simulink model "realtime_motor"  (R2024b)
settings: Solver=ode5  StartTime=0.0  StopTime=20  FixedStep=0.001  RelTol=1e-3
InitFcn:
  | Init
values from neighbouring files (symbols this model uses):
  Beq = (Beq_hat_pos + Beq_hat_neg)/2    [Parameters_estimation.m]    (also in Real_time_parameter_estimation.m = (data.Beq_hat_pos + data.Beq_hat_neg)/2; real-time-estimation.mat = 9.67900035512e-07)
  delta_est = 1/sqrt(2)    [Init.m]
  tau_sf = (abs(tau_sf_pos)+abs(tau_sf_neg))/2    [Parameters_estimation.m]    (also in Real_time_parameter_estimation.m = (abs(data.tau_sf_pos)+abs(data.tau_sf_neg))/2; real-time-estimation.mat = 0.00454084382337)
  wc = 2*pi*20    (= 125.663706144)    [Init.m]
undefined symbols (not defined in the file or in its folder): degs2rpm, gbox, Kd, Ki, Kp, mot, National_Instruments, PCI, rpm2degs, rpm2rads, sens, tl
libraries: sldrtlib x3, simulink x2
settings Model: SimulationMode=external  ExtModeTrigDuration=1000001  Creator=galeazzolu  LastModifiedBy=galeazzolu
settings DataIOCC: ReturnWorkspaceOutputs=off
settings HardwareCC: ProdBitPerLong=64  ProdHWDeviceType=Intel->x86-64 (Linux 64)
settings RTWCC: Description=Simulink Desktop Real-Time  SystemTargetFile=sldrt.tlc  TemplateMakefile=sldrt.tmf  RTWCompilerOptimization=on
settings CodeAppCC: MaxIdLength=95
settings SimulinkDesktopRealTimeCC: TargetLibSuffix=_sldrt.a  TargetPreCompLibLocation=C:\Program Files\MATLAB\R2024b\toolbox\sldrt\lib\win64  ParMdlRefBuildCompliant=on

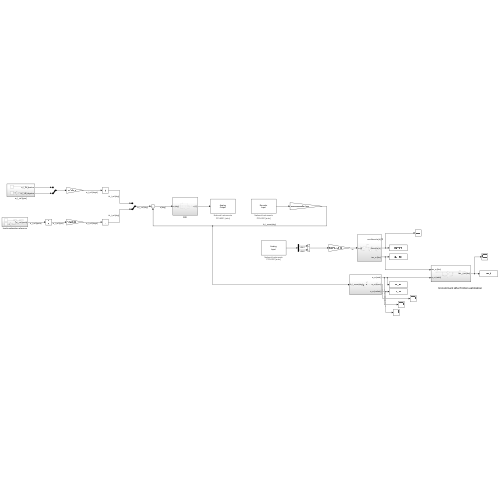
[thumbnail: Simulink's stored preview of the top-level diagram]
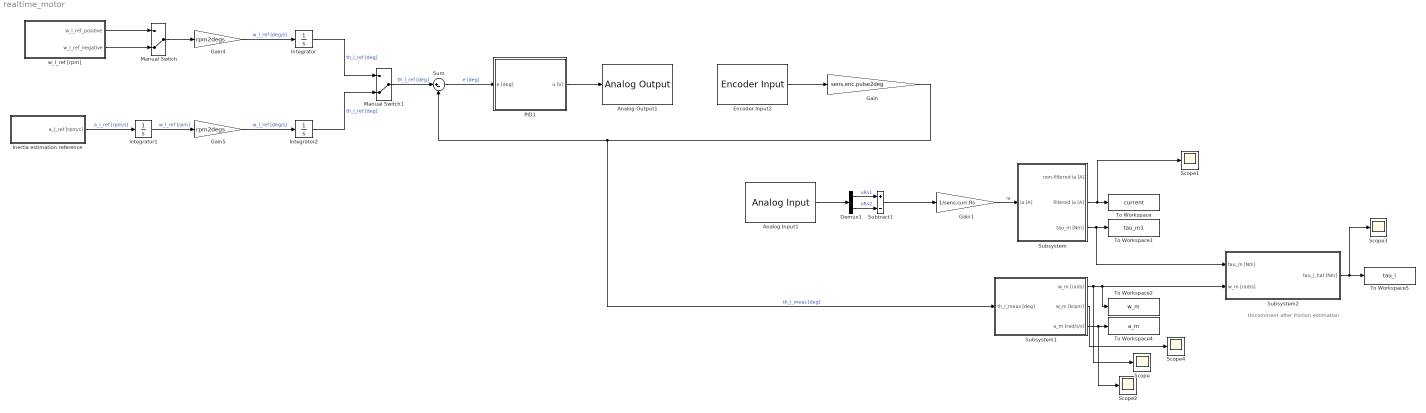
== system realtime_motor ==
  note: Uncomment after friction estimation
  Analog Input1 : sldrtlib/Analog Input  SampleTime=-1  MaxMissedTicks=10  ShowMissedTicks=off  YieldWhenWaiting=off  DrvName=National_Instruments/PCI-6221  DrvAddress=4294967295  DrvOptions=[0 0 0 2 0]  Channels=[1,2]  RangeMode=1  VoltRange=1  DataType=1
      settings: AttributesFormatString=National Instruments\nPCI-6221 [auto]
  Analog Output1 : sldrtlib/Analog Output  SampleTime=-1  MaxMissedTicks=10  ShowMissedTicks=off  YieldWhenWaiting=off  DrvName=National_Instruments/PCI-6221  DrvAddress=4294967295  DrvOptions=[0 0 0 2 0]  Channels=1  RangeMode=1  VoltRange=1  InitialValue=0  FinalValue=0
      settings: AttributesFormatString=National Instruments\nPCI-6221 [auto]
  Demux1 : Demux  Outputs=2
  Encoder Input2 : sldrtlib/Encoder Input  SampleTime=-1  MaxMissedTicks=10  ShowMissedTicks=off  YieldWhenWaiting=off  DrvName=National_Instruments/PCI-6221  DrvAddress=4294967295  DrvOptions=[0 0 0 2 0]  Channels=1  QuadMode=3  IndexPulse=1  InputFilter=Inf  DataType=1
      settings: AttributesFormatString=National Instruments\nPCI-6221 [auto]
  Gain : Gain  Gain=sens.enc.pulse2deg
  Gain1 : Gain  Gain=1/sens.curr.Rs
  Gain4 : Gain  Gain=rpm2degs
  Gain5 : Gain  Gain=rpm2degs
  Inertia estimation reference : Subsystem
  Integrator : Integrator
  Integrator1 : Integrator
  Integrator2 : Integrator
  Manual Switch : ManualSwitch  CurrentSetting=0
  Manual Switch1 : ManualSwitch  CurrentSetting=0
  PID1 : Subsystem
  Scope{,1..4} (5 alike) : Scope
  Subsystem : Subsystem
  Subsystem1 : Subsystem
  Subsystem2 : Subsystem
  Subtract1 : Sum  Inputs=+-
  Sum : Sum  Inputs=|+-
  To Workspace : ToWorkspace  VariableName=current  SaveFormat=Structure With Time  SampleTime=-1
  To Workspace1 : ToWorkspace  VariableName=tau_m1  SaveFormat=Structure With Time  SampleTime=-1
  To Workspace2 : ToWorkspace  VariableName=w_m  SaveFormat=Structure With Time  SampleTime=-1
  To Workspace4 : ToWorkspace  VariableName=a_m  SaveFormat=Structure With Time  SampleTime=-1
  To Workspace5 : ToWorkspace  VariableName=tau_i  SaveFormat=Structure With Time  SampleTime=-1
  w_l_ref [rpm] : Subsystem
  wires:
  Integrator1/1 -> Gain5/1  "w_l_ref [rpm]"
  w_l_ref [rpm]/1(w_l_ref_positive) -> Manual Switch/1
  Integrator2/1 -> Manual Switch1/2  "th_l_ref [deg]"
  Subsystem1/2(w_m [krpm]) -> Scope4/1
  Subsystem/2(filtered ia [A]) -> Scope1/1, To Workspace/1
  Manual Switch1/1 -> Sum/1  "th_l_ref [deg]"
  Sum/1 -> PID1/1(e [deg])  "e [deg]"
  PID1/1(u [V]) -> Analog Output1/1
  w_l_ref [rpm]/2(w_l_ref_negative) -> Manual Switch/2
  Gain/1 -> Subsystem1/1(th_l_meas [deg]), Sum/2  "th_l_meas [deg]"
  Demux1/1 -> Subtract1/1  "uRs1"
  Subsystem/3(tau_m [Nm]) -> Subsystem2/1(tau_m [Nm]), To Workspace1/1
  Gain4/1 -> Integrator/1  "w_l_ref [deg/s]"
  Gain1/1 -> Subsystem/1(ia [A])  "ia"
  Subsystem1/1(w_m [rads]) -> Subsystem2/2(w_m [rad/s]), To Workspace2/1, Scope/1
  Manual Switch/1 -> Gain4/1
  Demux1/2 -> Subtract1/2  "uRs2"
  Subsystem2/1(tau_i_hat [Nm]) -> Scope3/1, To Workspace5/1
  Integrator/1 -> Manual Switch1/1  "th_l_ref [deg]"
  Subtract1/1 -> Gain1/1
  Gain5/1 -> Integrator2/1  "w_l_ref [deg/s]"
  Inertia estimation reference/1(a_l_ref [rpm/s]) -> Integrator1/1  "a_l_ref [rpm/s]"
  Subsystem1/3(a_m [rad/s/s]) -> Scope2/1, To Workspace4/1
  Encoder Input2/1 -> Gain/1
  Analog Input1/1 -> Demux1/1

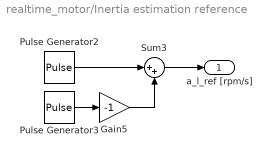
== system realtime_motor/Inertia estimation reference ==
  Gain5 : Gain  Gain=-1
  Pulse Generator2 : DiscretePulseGenerator  PulseType=Time based  Amplitude=450  PulseWidth=50
  Pulse Generator3 : DiscretePulseGenerator  PulseType=Time based  Amplitude=450  PulseWidth=50  PhaseDelay=1
  Sum3 : Sum  Inputs=|++
  a_l_ref [rpm/s] : Outport
  wires:
  Pulse Generator3/1 -> Gain5/1
  Pulse Generator2/1 -> Sum3/1
  Gain5/1 -> Sum3/2
  Sum3/1 -> a_l_ref [rpm/s]/1

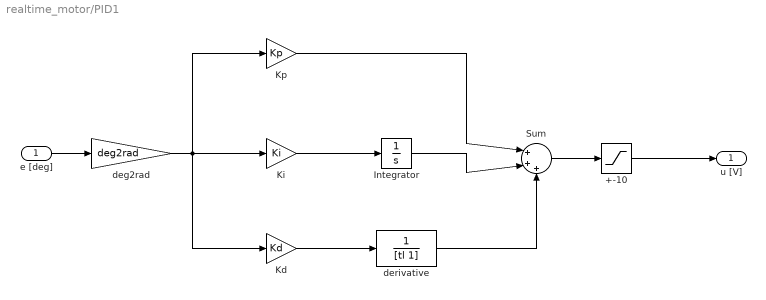
== system realtime_motor/PID1 ==
  e [deg] : Inport
  +-10 : Saturate  UpperLimit=10  LowerLimit=-10
  Integrator : Integrator
  Kd : Gain  Gain=Kd
  Ki : Gain  Gain=Ki
  Kp : Gain  Gain=Kp
  Sum : Sum  Inputs=|+++
  deg2rad : Gain  Gain=deg2rad
  derivative : TransferFcn  Denominator=[tl 1]
  u [V] : Outport
  wires:
  e [deg]/1 -> deg2rad/1
  deg2rad/1 -> Kd/1, Kp/1, Ki/1
  Ki/1 -> Integrator/1
  Kp/1 -> Sum/1
  Integrator/1 -> Sum/2
  Kd/1 -> derivative/1
  derivative/1 -> Sum/3
  Sum/1 -> +-10/1
  +-10/1 -> u [V]/1

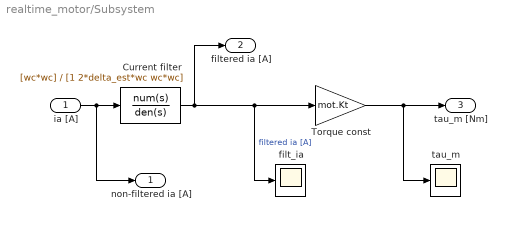
== system realtime_motor/Subsystem ==
  ia [A] : Inport
  " Current filter" : TransferFcn  Numerator=[wc*wc]  Denominator=[1 2*delta_est*wc wc*wc]
  Torque const : Gain  Gain=mot.Kt
  filt_ia : Scope
  tau_m : Scope
  non-filtered ia [A] : Outport
  filtered ia [A] : Outport  Port=2
  tau_m [Nm] : Outport  Port=3
  wires:
  " Current filter"/1 -> filtered ia [A]/1, filt_ia/1, Torque const/1  "filtered ia [A]"
  Torque const/1 -> tau_m [Nm]/1, tau_m/1
  ia [A]/1 -> non-filtered ia [A]/1, " Current filter"/1

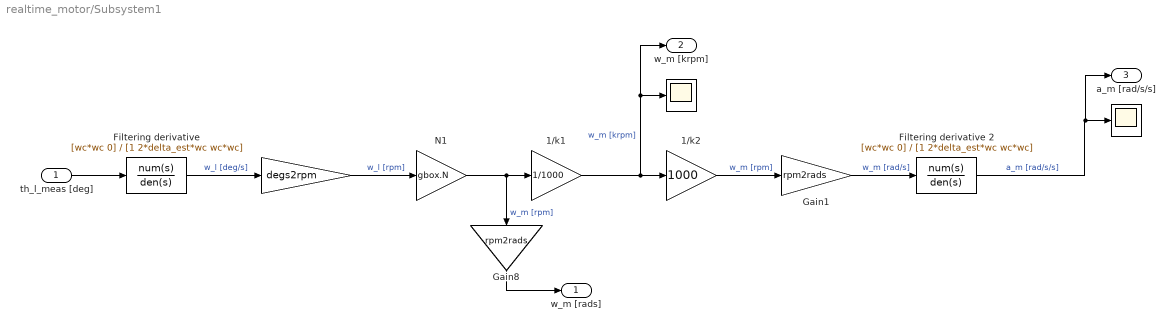
== system realtime_motor/Subsystem1 ==
  th_l_meas [deg] : Inport
  " " : Gain  Gain=degs2rpm
  "  " : Scope
  "    " : Scope
  1/k1 : Gain  Gain=1/1000
  1/k2 : Gain  Gain=1000
  Filtering derivative : TransferFcn  Numerator=[wc*wc 0]  Denominator=[1 2*delta_est*wc wc*wc]
  Filtering derivative 2 : TransferFcn  Numerator=[wc*wc 0]  Denominator=[1 2*delta_est*wc wc*wc]
  Gain1 : Gain  Gain=rpm2rads
  Gain8 : Gain  Gain=rpm2rads
  N1 : Gain  Gain=gbox.N
  w_m [rads] : Outport
  w_m [krpm] : Outport  Port=2
  a_m [rad/s/s] : Outport  Port=3
  wires:
  N1/1 -> Gain8/1, 1/k1/1  "w_m [rpm]"
  1/k1/1 -> "  "/1, w_m [krpm]/1, 1/k2/1  "w_m [krpm]"
  Gain8/1 -> w_m [rads]/1
  Filtering derivative/1 -> " "/1  "w_l [deg/s]"
  Filtering derivative 2/1 -> a_m [rad/s/s]/1, "    "/1  "a_m [rad/s/s]"
  " "/1 -> N1/1  "w_l [rpm]"
  th_l_meas [deg]/1 -> Filtering derivative/1
  1/k2/1 -> Gain1/1  "w_m [rpm]"
  Gain1/1 -> Filtering derivative 2/1  "w_m [rad/s]"

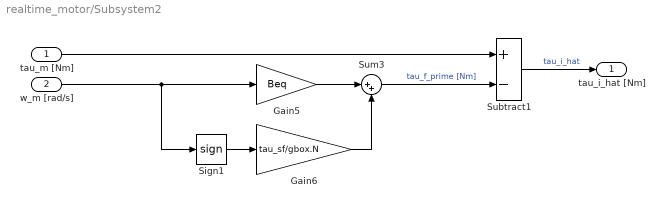
== system realtime_motor/Subsystem2 ==
  tau_m [Nm] : Inport
  w_m [rad/s] : Inport  Port=2
  Gain5 : Gain  Gain=Beq
  Gain6 : Gain  Gain=tau_sf/gbox.N
  Sign1 : Signum  ZeroCross=off
  Subtract1 : Sum  Inputs=+-
  Sum3 : Sum  Inputs=|++
  tau_i_hat [Nm] : Outport
  wires:
  Subtract1/1 -> tau_i_hat [Nm]/1  "tau_i_hat"
  tau_m [Nm]/1 -> Subtract1/1
  Gain5/1 -> Sum3/1
  Sum3/1 -> Subtract1/2  "tau_f_prime [Nm]"
  Sign1/1 -> Gain6/1
  Gain6/1 -> Sum3/2
  w_m [rad/s]/1 -> Sign1/1, Gain5/1

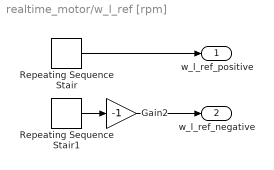
== system realtime_motor/w_l_ref [rpm] ==
  Gain2 : Gain  Gain=-1
  Repeating Sequence Stair : simulink/Sources/Repeating Sequence Stair  OutValues=[50 100 150 200 250 300 350 400 450 450].'  tsamp=5  OutMin=[]  OutMax=[]  OutDataTypeStr=double  OutputDataTypeScalingMode=double  OutDataType=fixdt(0,8)  ConRadixGroup=Best Precision: Vector-wise  OutScaling=2^-12
  Repeating Sequence Stair1 : simulink/Sources/Repeating Sequence Stair  OutValues=[50 100 150 200 250 300 350 400 450 450].'  tsamp=5  OutMin=[]  OutMax=[]  OutDataTypeStr=double  OutputDataTypeScalingMode=double  OutDataType=fixdt(0,8)  ConRadixGroup=Best Precision: Vector-wise  OutScaling=2^-12
  w_l_ref_positive : Outport
  w_l_ref_negative : Outport  Port=2
  wires:
  Repeating Sequence Stair1/1 -> Gain2/1
  Gain2/1 -> w_l_ref_negative/1
  Repeating Sequence Stair/1 -> w_l_ref_positive/1
